simulink model "wind_turbine_model"  (R2024a)
settings: Solver=VariableStepAuto  StartTime=0.0  StopTime=10.0  RelTol=1e-3
settings Model: Creator=Aman  LastModifiedBy=Aman

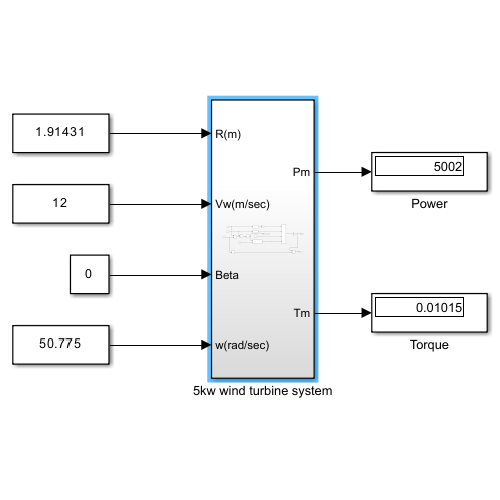
[thumbnail: Simulink's stored preview of the top-level diagram]
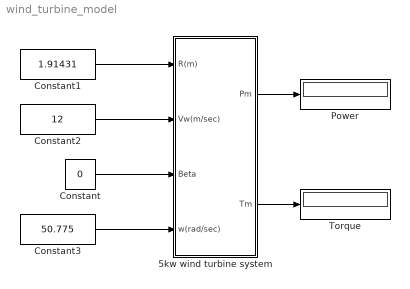
== system wind_turbine_model ==
  5kw wind turbine system : Subsystem
  Constant : Constant  Value=0
  Constant1 : Constant  Value=1.91431
  Constant2 : Constant  Value=12
  Constant3 : Constant  Value=50.775
  Power : Display
  Torque : Display
  wires:
  Constant/1 -> 5kw wind turbine system/3(Beta)
  Constant1/1 -> 5kw wind turbine system/1(R(m))
  Constant2/1 -> 5kw wind turbine system/2(Vw(m/sec))
  Constant3/1 -> 5kw wind turbine system/4(w(rad/sec))
  5kw wind turbine system/1(Pm) -> Power/1
  5kw wind turbine system/2(Tm) -> Torque/1

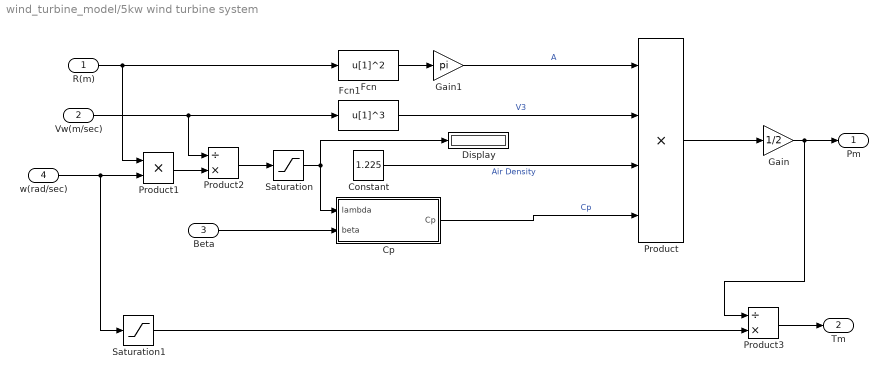
== system wind_turbine_model/5kw wind turbine system ==
  R(m) : Inport
  Vw(m/sec) : Inport  Port=2
  Beta : Inport  Port=3
  w(rad/sec) : Inport  Port=4
  Constant : Constant  Value=1.225
  Cp : Subsystem
  Display : Display
  Fcn : Fcn  Expr=u[1]^2
  Fcn1 : Fcn  Expr=u[1]^3
  Gain : Gain  Gain=1/2
  Gain1 : Gain  Gain=pi
  Product : Product  Inputs=4
  Product1 : Product
  Product2 : Product  Inputs=/*
  Product3 : Product  Inputs=/*
  Saturation : Saturate  UpperLimit=inf  LowerLimit=1e-6
  Saturation1 : Saturate  UpperLimit=inf  LowerLimit=1e-6
  Pm : Outport
  Tm : Outport  Port=2
  wires:
  Product/1 -> Gain/1
  Gain/1 -> Product3/1, Pm/1
  Gain1/1 -> Product/1  "A"
  Fcn1/1 -> Product/2  "V3"
  Constant/1 -> Product/3  "Air Density"
  Cp/1(Cp) -> Product/4  "Cp"
  R(m)/1 -> Product1/1, Fcn/1
  Fcn/1 -> Gain1/1
  Vw(m/sec)/1 -> Product2/1, Fcn1/1
  w(rad/sec)/1 -> Saturation1/1, Product1/2
  Product1/1 -> Product2/2
  Product2/1 -> Saturation/1
  Saturation/1 -> Display/1, Cp/1(lambda)
  Beta/1 -> Cp/2(beta)
  Saturation1/1 -> Product3/2
  Product3/1 -> Tm/1

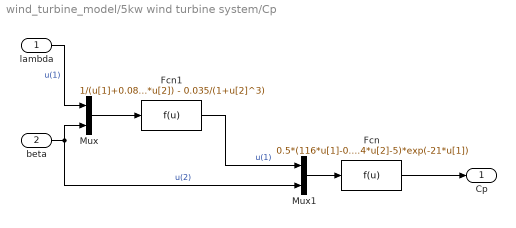
== system wind_turbine_model/5kw wind turbine system/Cp ==
  lambda : Inport
  beta : Inport  Port=2
  Fcn : Fcn  Expr=0.5*(116*u[1]-0.4*u[2]-5)*exp(-21*u[1])
  Fcn1 : Fcn  Expr=1/(u[1]+0.08*u[2]) - 0.035/(1+u[2]^3)
  Mux : Mux  Inputs=3
  Mux1 : Mux  Inputs=2
  Cp : Outport
  wires:
  Fcn/1 -> Cp/1
  lambda/1 -> Mux/1  "u(1)"
  Mux1/1 -> Fcn/1
  Fcn1/1 -> Mux1/1  "u(1)"
  beta/1 -> Mux1/2, Mux/3  "u(2)"
  Mux/1 -> Fcn1/1
